simulink model "FireFighter_original"  (R2014a)
settings: Solver=ode45  StartTime=0.0  StopTime=150  RelTol=1e-3
undefined symbols (not defined in the file): DiscIntNeverNeededParam, sigbuilder_block
libraries: simulink x68
(part 2 of 6)

== system FireFighter_original/FF_Signals4/Environment1 ==
  note: F_hill
  note: F_eng_resistance
  note: F_resistance
  note: F_eng
  note: position
  note: speed
  note: slope
  gas : Inport
  brake : Inport  Port=2
  1/mass2 : Gain  Gain=0.001
  Discrete-Time Integrator : DiscreteIntegrator  SampleTime=-1  ICPrevOutput=DiscIntNeverNeededParam  ICPrevScaledInput=DiscIntNeverNeededParam
  Discrete-Time Integrator1 : DiscreteIntegrator  SampleTime=-1  ICPrevOutput=DiscIntNeverNeededParam  ICPrevScaledInput=DiscIntNeverNeededParam
  Fast - to - Slow : RateTransition  OutPortSampleTimeMultiple=0.05  OutPortSampleTime=0.1
  "Fast - to - Slow1 " : RateTransition  OutPortSampleTimeMultiple=0.05  OutPortSampleTime=0.1
  Fcn : Fcn  Expr=u(1)/0.005
  Gain1 : Gain  Gain=0.0005
  Max Torque by rpm6 : Lookup_n-D  NumberOfTableDimensions=1  BreakpointsForDimension1=[0;8;20;28;40;60;80;100;120;140;160;180;200]  Table=[165;180;180;170;170;150;115;97;80;70;60;50;40]  RndMeth=Simplest  InputSameDT=on
  Max Torque by rpm9 : Lookup_n-D  NumberOfTableDimensions=1  BreakpointsForDimension1=[0:1000:15000]  Table=[0;pi/60;pi/30;pi/20;pi/15;pi/12;0;0;-pi/18;-pi/36;0;0;0;0;0;0]  RndMeth=Simplest  InputSameDT=on
  Product1 : Product  RndMeth=Zero
  Scope{2..3,6..15,27} (13 alike) : Scope
      Scope10 settings: SaveName=ScopeData23
      Scope11 settings: TimeRange=10  YMin=-50  YMax=300  SaveName=ScopeData26
      Scope12 settings: SaveName=ScopeData32
      Scope13 settings: SaveName=ScopeData33
      Scope14 settings: SaveName=ScopeData15
      Scope15 settings: SaveName=ScopeData19
      Scope2 settings: TimeRange=10  YMin=-50  YMax=300  SaveName=ScopeData6
      Scope27 settings: TimeRange=10  YMin=-50  YMax=300  SaveName=ScopeData49
      Scope3 settings: SaveName=ScopeData8
      Scope6 settings: TimeRange=100  YMin=89.9904  YMax=89.9913  SaveName=ScopeData16
      Scope7 settings: SaveName=ScopeData10
      Scope8 settings: SaveName=ScopeData21
      Scope9 settings: SaveName=ScopeData22
  Slow - to - Fast : RateTransition  OutPortSampleTimeMultiple=0.05  OutPortSampleTime=0.05
  Step1 : Step  Time=0  After=700
  Sum1 : Sum  Inputs=|++
  Sum4 : Sum  Inputs=|+---
  Trigonometric Function1 : Trigonometry
  brake force1 : Gain  Gain=10000
  g1 : Gain  Gain=9.80665
  mass3 : Gain  Gain=1000
  pos : Outport
  wires:
  Step1/1 -> Sum1/2
  Product1/1 -> Fcn/1
  brake force1/1 -> Scope12/1, Sum4/2
  Sum4/1 -> Scope7/1, 1/mass2/1
  1/mass2/1 -> Discrete-Time Integrator/1, Scope8/1
  Gain1/1 -> Scope13/1, Sum4/3
  gas/1 -> Scope14/1, Fast - to - Slow/1
  brake/1 -> Scope15/1, "Fast - to - Slow1 "/1
  Discrete-Time Integrator/1 -> Max Torque by rpm6/1, Gain1/1, Discrete-Time Integrator1/1, Scope6/1
  Discrete-Time Integrator1/1 -> Max Torque by rpm9/1, Scope2/1, Sum1/1
  Max Torque by rpm9/1 -> Trigonometric Function1/1
  g1/1 -> mass3/1
  Trigonometric Function1/1 -> g1/1
  mass3/1 -> Sum4/4, Scope3/1
  Fcn/1 -> Scope10/1, Sum4/1
  Fast - to - Slow/1 -> Product1/2
  "Fast - to - Slow1 "/1 -> brake force1/1
  Sum1/1 -> Scope27/1, Slow - to - Fast/1
  Slow - to - Fast/1 -> pos/1, Scope11/1
  Max Torque by rpm6/1 -> Product1/1, Scope9/1

== system FireFighter_original/FF_Signals4/FireFighter1 ==
  note: current speed
  note: speed=90
  pos : Inport
  Constant : Constant  Value=0
  Constant2 : Constant  Value=90
  Discrete Derivative : simulink/Discrete/Discrete Derivative  gainval=1.0  ICPrevScaledInput=0.0  InputProcessing=Inherited  OutMin=[]  OutMax=[]  OutDataType=fixdt(1, 16)  OutScaling=2^-10  DoSatur=off
  Discrete PID Controller : simulink/Continuous/PID Controller  Controller=PI  TimeDomain=Discrete-time  SampleTime=-1  IntegratorMethod=Forward Euler  FilterMethod=Forward Euler  Form=Parallel  P=0.05  I=0.000228325  D=0  N=100  InitialConditionSource=internal  InitialConditionForIntegrator=0  InitialConditionForFilter=0  ExternalReset=none  LimitOutput=on  UpperSaturationLimit=1  LowerSaturationLimit=-1  LinearizeAsGain=off  AntiWindupMode=back-calculation  Kb=0.01  TrackingMode=off  Kt=1  PParamMin=[]  PParamMax=[]  IParamMin=[]  IParamMax=[]  DParamMin=[]  DParamMax=[]  NParamMin=[]  NParamMax=[]  KbParamMin=[]  KbParamMax=[]  KtParamMin=[]  KtParamMax=[]  POutMin=[]  POutMax=[]  IOutMin=[]  IOutMax=[]  DOutMin=[]  DOutMax=[]  NOutMin=[]  NOutMax=[]  KbOutMin=[]  KbOutMax=[]  KtOutMin=[]  KtOutMax=[]  IntegratorOutMin=[]  IntegratorOutMax=[]  FilterOutMin=[]  FilterOutMax=[]  SumOutMin=[]  SumOutMax=[]  SumI1OutMin=[]  SumI1OutMax=[]  SumI2OutMin=[]  SumI2OutMax=[]  SumI3OutMin=[]  SumI3OutMax=[]  SumDOutMin=[]  SumDOutMax=[]  SaturationOutMin=[]  SaturationOutMax=[]  IntegratorContinuousStateAttributes=''  IntegratorStateMustResolveToSignalObject=off  IntegratorRTWStateStorageClass=Auto  FilterContinuousStateAttributes=''  FilterStateMustResolveToSignalObject=off  FilterRTWStateStorageClass=Auto
  Fast - to -Slow : RateTransition  OutPortSampleTimeMultiple=0.05  OutPortSampleTime=0.1
  Gain : Gain  Gain=50
  Gain1 : Gain  Gain=-1
  Scope{1..2,4..9,11..13} (11 alike) : Scope
      Scope1 settings: TimeRange=100  YMin=90  YMax=130
      Scope11 settings: YMin=-300  YMax=300  SaveName=ScopeData28
      Scope12 settings: YMin=-300  YMax=300  SaveName=ScopeData30
      Scope13 settings: SaveName=ScopeData31
      Scope2 settings: YMin=-300  YMax=300  SaveName=ScopeData2
      Scope4 settings: YMin=-300  YMax=300  SaveName=ScopeData17
      Scope5 settings: SaveName=ScopeData20
      Scope6 settings: YMin=-300  YMax=300  SaveName=ScopeData18
      Scope7 settings: YMin=-300  YMax=300  SaveName=ScopeData24
      Scope8 settings: TimeRange=10  SaveName=ScopeData25
      Scope9 settings: SaveName=ScopeData38
  Signal Builder : Subsystem  Tag=STV Subsys  LoadFcn=sigbuilder_block('load');  StartFcn=sigbuilder_block('start');  StopFcn=sigbuilder_block('stop');  ClipboardFcn=sigbuilder_block('clipboard');  mask(Sigbuilder block){}
      mask help: Simulink:masks:SigbuilderBlock_MD
      mask init:
      | if ~strcmp(get_param(bdroot(gcbh),'SimulationStatus'),'stopped') tuvar = sigbuilder_block('maskInit'); end
      settings: CopyFcn=sigbuilder_block('copy');  DeleteFcn=sigbuilder_block('delete');  ModelCloseFcn=sigbuilder_block('modelClose');  PreSaveFcn=sigbuilder_block('preSave');  PauseFcn=sigbuilder_block('pause');  ContinueFcn=sigbuilder_block('continue');  NameChangeFcn=sigbuilder_block('namechange');  OpenFcn=sigbuilder_block('open',[359.25 300.75 550.5 399.75 ]);  CloseFcn=sigbuilder_block('close');
      mask Display: plot(0, 0, 100, 100,[2, 2, 32, 32, 2], [68, 8, 8, 68, 68],[32, 2], [38, 38], [32, 19, 2],[53, 60, 44], [32, 17, 17, 2],[16, 16, 31, 31]);txt = getActiveGroup(gcbh);text(2, 100, txt,'verticalAlignment', 'top');
  Slow - to - Fast : RateTransition  OutPortSampleTimeMultiple=0.05  OutPortSampleTime=0.05
  Slow - to - Fast1 : RateTransition  OutPortSampleTimeMultiple=0.05  OutPortSampleTime=0.05
  Sum : Sum  Inputs=|+-
  Sum1 : Sum  Inputs=|++
  Switch : Switch
  Switch1 : Switch
  Zero-Order Hold : ZeroOrderHold  SampleTime=0.1
  gas : Outport
  brake : Outport  Port=2
  wires:
  Discrete Derivative/1 -> Scope8/1, Sum/2
  Signal Builder/1(Signal 1) -> Gain/1
  Gain/1 -> Zero-Order Hold/1
  Constant2/1 -> Sum1/2
  Discrete PID Controller/1 -> Scope2/1, Scope7/1, Switch/1, Switch/2, Switch1/2, Gain1/1
  Gain1/1 -> Switch1/3
  Switch/1 -> Slow - to - Fast/1, Scope4/1
  Constant/1 -> Switch/3, Switch1/1
  Switch1/1 -> Slow - to - Fast1/1, Scope6/1
  pos/1 -> Scope13/1, Fast - to -Slow/1
  Sum/1 -> Discrete PID Controller/1, Scope9/1
  Fast - to -Slow/1 -> Discrete Derivative/1, Scope5/1
  Slow - to - Fast/1 -> Scope11/1, gas/1
  Slow - to - Fast1/1 -> Scope12/1, brake/1
  Sum1/1 -> Scope1/1, Sum/1
  Zero-Order Hold/1 -> Sum1/1

== system FireFighter_original/FF_Signals4/Inaccuracy ==
  note: max
  pos_init : Inport
  hold : Inport  Port=2
  Mux29 : Mux  Inputs=2
  Product : Product
  Product1 : Product
  Scope{1..3,5..7,9} (7 alike) : Scope
      Scope1 settings: SaveName=ScopeData29
      Scope2 settings: SaveName=ScopeData43
      Scope3 settings: SaveName=ScopeData35
      Scope5 settings: SaveName=ScopeData46
      Scope6 settings: SaveName=ScopeData48
      Scope7 settings: TimeRange=150  SaveName=ScopeData57
      Scope9 settings: SaveName=ScopeData44
  Subsystem1 : Subsystem
  Subsystem2 : Subsystem
  Subtract1 : Sum  Inputs=-+
  result : Outport
  wires:
  Subsystem2/1(min) -> Product/1, Scope2/1  "min"
  pos_init/1 -> Subsystem1/1(pos_init), Subsystem2/1(pos_init), Scope1/1
  Mux29/1 -> result/1
  Subsystem1/1(max) -> Product1/2, Scope9/1
  Product/1 -> Mux29/1, Scope6/1, Subtract1/1
  Product1/1 -> Scope5/1, Mux29/2, Subtract1/2
  hold/1 -> Subsystem2/2(hold), Scope3/1, Product/2, Product1/1, Subsystem1/2(hold)
  Subtract1/1 -> Scope7/1

== system FireFighter_original/FF_Signals4/Inaccuracy1 ==
  note: max
  Hpos_inits : Inport
  holds : Inport  Port=2
  Mux29 : Mux  Inputs=2
  Product : Product
  Product1 : Product
  Scope{1..3,5..7,9} (7 alike) : Scope
      Scope1 settings: SaveName=ScopeData29
      Scope2 settings: SaveName=ScopeData43
      Scope3 settings: SaveName=ScopeData35
      Scope5 settings: SaveName=ScopeData46
      Scope6 settings: SaveName=ScopeData48
      Scope7 settings: TimeRange=150  SaveName=ScopeData57
      Scope9 settings: SaveName=ScopeData44
  Subsystem1 : Subsystem
  Subsystem2 : Subsystem
  Subtract1 : Sum  Inputs=-+
  result : Outport
  wires:
  Subsystem2/1(min) -> Product/1, Scope2/1  "min"
  Hpos_inits/1 -> Subsystem1/1(pos_init), Subsystem2/1(pos_init), Scope1/1
  Mux29/1 -> result/1
  Subsystem1/1(max) -> Product1/2, Scope9/1
  Product/1 -> Mux29/1, Scope6/1, Subtract1/1
  Product1/1 -> Scope5/1, Mux29/2, Subtract1/2
  holds/1 -> Subsystem2/2(hold), Scope3/1, Product/2, Product1/1, Subsystem1/2(hold)
  Subtract1/1 -> Scope7/1

== system FireFighter_original/FF_Signals4/Inaccuracy2 ==
  note: max
  Hpos_inits : Inport
  holds : Inport  Port=2
  Mux29 : Mux  Inputs=2
  Product : Product
  Product1 : Product
  Scope{1..3,5..7,9} (7 alike) : Scope
      Scope1 settings: SaveName=ScopeData29
      Scope2 settings: SaveName=ScopeData43
      Scope3 settings: SaveName=ScopeData35
      Scope5 settings: SaveName=ScopeData46
      Scope6 settings: SaveName=ScopeData48
      Scope7 settings: TimeRange=150  SaveName=ScopeData57
      Scope9 settings: SaveName=ScopeData44
  Subsystem1 : Subsystem
  Subsystem2 : Subsystem
  Subtract1 : Sum  Inputs=-+
  result : Outport
  wires:
  Subsystem2/1(min) -> Product/1, Scope2/1  "min"
  Hpos_inits/1 -> Subsystem1/1(pos_init), Subsystem2/1(pos_init), Scope1/1
  Mux29/1 -> result/1
  Subsystem1/1(max) -> Product1/2, Scope9/1
  Product/1 -> Mux29/1, Scope6/1, Subtract1/1
  Product1/1 -> Scope5/1, Mux29/2, Subtract1/2
  holds/1 -> Subsystem2/2(hold), Scope3/1, Product/2, Product1/1, Subsystem1/2(hold)
  Subtract1/1 -> Scope7/1

== system FireFighter_original/FF_Signals4/START THE MESSION2 ==
  Demux : Demux  Tag=STV Demux  Outputs=1
  FromWs : FromWorkspace  Tag=STV FromWs  VariableName=tuvar  SampleTime=0
      SigBuilderData=|
      | common.afterFinalStr = 'Extrapolate'
      | common.sampleTime = 0
      | dataSet.timeRange = [0 1000]
      | dataSet.name = 'Group 1'
      | sbobj.Groups.Name = 'Group 1'
      | sbobj.Groups.Signals.Name = 'SWITCH'
      | sbobj.Groups.Signals.XData = [0 20 20 1000]
      | sbobj.Groups.Signals.YData = [0 0 1 1]
      | sbobj.Groups.TimeRange = [0 1000]
  SWITCH : Outport  Tag=STV Outport
  wires:
  FromWs/1 -> Demux/1
  Demux/1 -> SWITCH/1

== system FireFighter_original/Inaccuracy/Subsystem1 ==
  pos_init : Inport
  hold : Inport  Port=2
  Environment : Subsystem
  FireFighter : Subsystem
  max : Outport
  wires:
  Environment/1(pos) -> FireFighter/1(pos), max/1
  FireFighter/1(gas) -> Environment/1(gas)
  FireFighter/2(brake) -> Environment/2(brake)
  pos_init/1 -> Environment/3(pos_init)
  hold/1 -> Environment/4(hold)

== system FireFighter_original/Inaccuracy/Subsystem2 ==
  pos_init : Inport
  hold : Inport  Port=2
  Environment : Subsystem
  FireFighter : Subsystem
  min : Outport
  wires:
  Environment/1(pos) -> FireFighter/1(pos), min/1
  FireFighter/1(gas) -> Environment/1(gas)
  FireFighter/2(brake) -> Environment/2(brake)
  pos_init/1 -> Environment/3(pos_init)
  hold/1 -> Environment/4(hold)

== system FireFighter_original/FF_Signals/FireFighter/Signal Builder ==
  Demux : Demux  Tag=STV Demux  Outputs=1
  FromWs : FromWorkspace  Tag=STV FromWs  VariableName=tuvar  SampleTime=0
      SigBuilderData=|
      | common.afterFinalStr = 'Extrapolate'
      | common.sampleTime = 0
      | dataSet.timeRange = [0 100]
      | dataSet.name = 'Group 1'
      | sbobj.Groups.Name = 'Group 1'
      | sbobj.Groups.Signals.Name = 'Signal 1'
      | sbobj.Groups.Signals.XData = [0 30 40 50 70 100]
      | sbobj.Groups.Signals.YData = [0 0 0.6 -0.405 0 0]
      | sbobj.Groups.TimeRange = [0 100]
  Signal 1 : Outport  Tag=STV Outport
  wires:
  Demux/1 -> Signal 1/1
  FromWs/1 -> Demux/1

== system FireFighter_original/FF_Signals1/FireFighter1/Signal Builder ==
  Demux : Demux  Tag=STV Demux  Outputs=1
  FromWs : FromWorkspace  Tag=STV FromWs  VariableName=tuvar  SampleTime=0
      SigBuilderData=|
      | common.afterFinalStr = 'Extrapolate'
      | common.sampleTime = 0
      | dataSet.timeRange = [0 100]
      | dataSet.name = 'Group 1'
      | sbobj.Groups.Name = 'Group 1'
      | sbobj.Groups.Signals.Name = 'Signal 1'
      | sbobj.Groups.Signals.XData = [0 30 40 50 70 100]
      | sbobj.Groups.Signals.YData = [0 0 0.6 -0.405 0 0]
      | sbobj.Groups.TimeRange = [0 100]
  Signal 1 : Outport  Tag=STV Outport
  wires:
  Demux/1 -> Signal 1/1
  FromWs/1 -> Demux/1

== system FireFighter_original/FF_Signals1/Inaccuracy/Subsystem1 ==
  pos_init : Inport
  hold : Inport  Port=2
  Environment : Subsystem
  FireFighter : Subsystem
  max : Outport
  wires:
  Environment/1(pos) -> FireFighter/1(pos), max/1
  FireFighter/1(gas) -> Environment/1(gas)
  FireFighter/2(brake) -> Environment/2(brake)
  pos_init/1 -> Environment/3(pos_init)
  hold/1 -> Environment/4(hold)

== system FireFighter_original/FF_Signals1/Inaccuracy/Subsystem2 ==
  pos_init : Inport
  hold : Inport  Port=2
  Environment : Subsystem
  FireFighter : Subsystem
  min : Outport
  wires:
  Environment/1(pos) -> FireFighter/1(pos), min/1
  FireFighter/1(gas) -> Environment/1(gas)
  FireFighter/2(brake) -> Environment/2(brake)
  pos_init/1 -> Environment/3(pos_init)
  hold/1 -> Environment/4(hold)

== system FireFighter_original/FF_Signals1/Inaccuracy1/Subsystem1 ==
  pos_init : Inport
  hold : Inport  Port=2
  Environment : Subsystem
  FireFighter : Subsystem
  max : Outport
  wires:
  Environment/1(pos) -> FireFighter/1(pos), max/1
  FireFighter/1(gas) -> Environment/1(gas)
  FireFighter/2(brake) -> Environment/2(brake)
  pos_init/1 -> Environment/3(pos_init)
  hold/1 -> Environment/4(hold)

== system FireFighter_original/FF_Signals1/Inaccuracy1/Subsystem2 ==
  pos_init : Inport
  hold : Inport  Port=2
  Environment : Subsystem
  FireFighter : Subsystem
  min : Outport
  wires:
  Environment/1(pos) -> FireFighter/1(pos), min/1
  FireFighter/1(gas) -> Environment/1(gas)
  FireFighter/2(brake) -> Environment/2(brake)
  pos_init/1 -> Environment/3(pos_init)
  hold/1 -> Environment/4(hold)

== system FireFighter_original/FF_Signals1/Inaccuracy2/Subsystem1 ==
  pos_init : Inport
  hold : Inport  Port=2
  Environment : Subsystem
  FireFighter : Subsystem
  max : Outport
  wires:
  Environment/1(pos) -> FireFighter/1(pos), max/1
  FireFighter/1(gas) -> Environment/1(gas)
  FireFighter/2(brake) -> Environment/2(brake)
  pos_init/1 -> Environment/3(pos_init)
  hold/1 -> Environment/4(hold)

== system FireFighter_original/FF_Signals1/Inaccuracy2/Subsystem2 ==
  pos_init : Inport
  hold : Inport  Port=2
  Environment : Subsystem
  FireFighter : Subsystem
  min : Outport
  wires:
  Environment/1(pos) -> FireFighter/1(pos), min/1
  FireFighter/1(gas) -> Environment/1(gas)
  FireFighter/2(brake) -> Environment/2(brake)
  pos_init/1 -> Environment/3(pos_init)
  hold/1 -> Environment/4(hold)

== system FireFighter_original/FF_Signals2/FireFighter1/Signal Builder ==
  Demux : Demux  Tag=STV Demux  Outputs=1
  FromWs : FromWorkspace  Tag=STV FromWs  VariableName=tuvar  SampleTime=0
      SigBuilderData=|
      | common.afterFinalStr = 'Extrapolate'
      | common.sampleTime = 0
      | dataSet.timeRange = [0 100]
      | dataSet.name = 'Group 1'
      | sbobj.Groups.Name = 'Group 1'
      | sbobj.Groups.Signals.Name = 'Signal 1'
      | sbobj.Groups.Signals.XData = [0 30 40 50 70 100]
      | sbobj.Groups.Signals.YData = [0 0 0.6 -0.405 0 0]
      | sbobj.Groups.TimeRange = [0 100]
  Signal 1 : Outport  Tag=STV Outport
  wires:
  Demux/1 -> Signal 1/1
  FromWs/1 -> Demux/1

== system FireFighter_original/FF_Signals2/Inaccuracy/Subsystem1 ==
  pos_init : Inport
  hold : Inport  Port=2
  Environment : Subsystem
  FireFighter : Subsystem
  max : Outport
  wires:
  Environment/1(pos) -> FireFighter/1(pos), max/1
  FireFighter/1(gas) -> Environment/1(gas)
  FireFighter/2(brake) -> Environment/2(brake)
  pos_init/1 -> Environment/3(pos_init)
  hold/1 -> Environment/4(hold)

== system FireFighter_original/FF_Signals2/Inaccuracy/Subsystem2 ==
  pos_init : Inport
  hold : Inport  Port=2
  Environment : Subsystem
  FireFighter : Subsystem
  min : Outport
  wires:
  Environment/1(pos) -> FireFighter/1(pos), min/1
  FireFighter/1(gas) -> Environment/1(gas)
  FireFighter/2(brake) -> Environment/2(brake)
  pos_init/1 -> Environment/3(pos_init)
  hold/1 -> Environment/4(hold)

== system FireFighter_original/FF_Signals2/Inaccuracy1/Subsystem1 ==
  pos_init : Inport
  hold : Inport  Port=2
  Environment : Subsystem
  FireFighter : Subsystem
  max : Outport
  wires:
  Environment/1(pos) -> FireFighter/1(pos), max/1
  FireFighter/1(gas) -> Environment/1(gas)
  FireFighter/2(brake) -> Environment/2(brake)
  pos_init/1 -> Environment/3(pos_init)
  hold/1 -> Environment/4(hold)

== system FireFighter_original/FF_Signals2/Inaccuracy1/Subsystem2 ==
  pos_init : Inport
  hold : Inport  Port=2
  Environment : Subsystem
  FireFighter : Subsystem
  min : Outport
  wires:
  Environment/1(pos) -> FireFighter/1(pos), min/1
  FireFighter/1(gas) -> Environment/1(gas)
  FireFighter/2(brake) -> Environment/2(brake)
  pos_init/1 -> Environment/3(pos_init)
  hold/1 -> Environment/4(hold)

== system FireFighter_original/FF_Signals2/Inaccuracy2/Subsystem1 ==
  pos_init : Inport
  hold : Inport  Port=2
  Environment : Subsystem
  FireFighter : Subsystem
  max : Outport
  wires:
  Environment/1(pos) -> FireFighter/1(pos), max/1
  FireFighter/1(gas) -> Environment/1(gas)
  FireFighter/2(brake) -> Environment/2(brake)
  pos_init/1 -> Environment/3(pos_init)
  hold/1 -> Environment/4(hold)

== system FireFighter_original/FF_Signals2/Inaccuracy2/Subsystem2 ==
  pos_init : Inport
  hold : Inport  Port=2
  Environment : Subsystem
  FireFighter : Subsystem
  min : Outport
  wires:
  Environment/1(pos) -> FireFighter/1(pos), min/1
  FireFighter/1(gas) -> Environment/1(gas)
  FireFighter/2(brake) -> Environment/2(brake)
  pos_init/1 -> Environment/3(pos_init)
  hold/1 -> Environment/4(hold)

== system FireFighter_original/FF_Signals4/FireFighter1/Signal Builder ==
  Demux : Demux  Tag=STV Demux  Outputs=1
  FromWs : FromWorkspace  Tag=STV FromWs  VariableName=tuvar  SampleTime=0
      SigBuilderData=|
      | common.afterFinalStr = 'Extrapolate'
      | common.sampleTime = 0
      | dataSet.timeRange = [0 100]
      | dataSet.name = 'Group 1'
      | sbobj.Groups.Name = 'Group 1'
      | sbobj.Groups.Signals.Name = 'Signal 1'
      | sbobj.Groups.Signals.XData = [0 30 40 50 70 100]
      | sbobj.Groups.Signals.YData = [0 0 0.6 -0.405 0 0]
      | sbobj.Groups.TimeRange = [0 100]
  Signal 1 : Outport  Tag=STV Outport
  wires:
  Demux/1 -> Signal 1/1
  FromWs/1 -> Demux/1

== system FireFighter_original/FF_Signals4/Inaccuracy/Subsystem1 ==
  pos_init : Inport
  hold : Inport  Port=2
  Environment : Subsystem
  FireFighter : Subsystem
  max : Outport
  wires:
  Environment/1(pos) -> FireFighter/1(pos), max/1
  FireFighter/1(gas) -> Environment/1(gas)
  FireFighter/2(brake) -> Environment/2(brake)
  pos_init/1 -> Environment/3(pos_init)
  hold/1 -> Environment/4(hold)

== system FireFighter_original/FF_Signals4/Inaccuracy/Subsystem2 ==
  pos_init : Inport
  hold : Inport  Port=2
  Environment : Subsystem
  FireFighter : Subsystem
  min : Outport
  wires:
  Environment/1(pos) -> FireFighter/1(pos), min/1
  FireFighter/1(gas) -> Environment/1(gas)
  FireFighter/2(brake) -> Environment/2(brake)
  pos_init/1 -> Environment/3(pos_init)
  hold/1 -> Environment/4(hold)

== system FireFighter_original/FF_Signals4/Inaccuracy1/Subsystem1 ==
  pos_init : Inport
  hold : Inport  Port=2
  Environment : Subsystem
  FireFighter : Subsystem
  max : Outport
  wires:
  Environment/1(pos) -> FireFighter/1(pos), max/1
  FireFighter/1(gas) -> Environment/1(gas)
  FireFighter/2(brake) -> Environment/2(brake)
  pos_init/1 -> Environment/3(pos_init)
  hold/1 -> Environment/4(hold)

== system FireFighter_original/FF_Signals4/Inaccuracy1/Subsystem2 ==
  pos_init : Inport
  hold : Inport  Port=2
  Environment : Subsystem
  FireFighter : Subsystem
  min : Outport
  wires:
  Environment/1(pos) -> FireFighter/1(pos), min/1
  FireFighter/1(gas) -> Environment/1(gas)
  FireFighter/2(brake) -> Environment/2(brake)
  pos_init/1 -> Environment/3(pos_init)
  hold/1 -> Environment/4(hold)

== system FireFighter_original/FF_Signals4/Inaccuracy2/Subsystem1 ==
  pos_init : Inport
  hold : Inport  Port=2
  Environment : Subsystem
  FireFighter : Subsystem
  max : Outport
  wires:
  Environment/1(pos) -> FireFighter/1(pos), max/1
  FireFighter/1(gas) -> Environment/1(gas)
  FireFighter/2(brake) -> Environment/2(brake)
  pos_init/1 -> Environment/3(pos_init)
  hold/1 -> Environment/4(hold)

== system FireFighter_original/FF_Signals4/Inaccuracy2/Subsystem2 ==
  pos_init : Inport
  hold : Inport  Port=2
  Environment : Subsystem
  FireFighter : Subsystem
  min : Outport
  wires:
  Environment/1(pos) -> FireFighter/1(pos), min/1
  FireFighter/1(gas) -> Environment/1(gas)
  FireFighter/2(brake) -> Environment/2(brake)
  pos_init/1 -> Environment/3(pos_init)
  hold/1 -> Environment/4(hold)

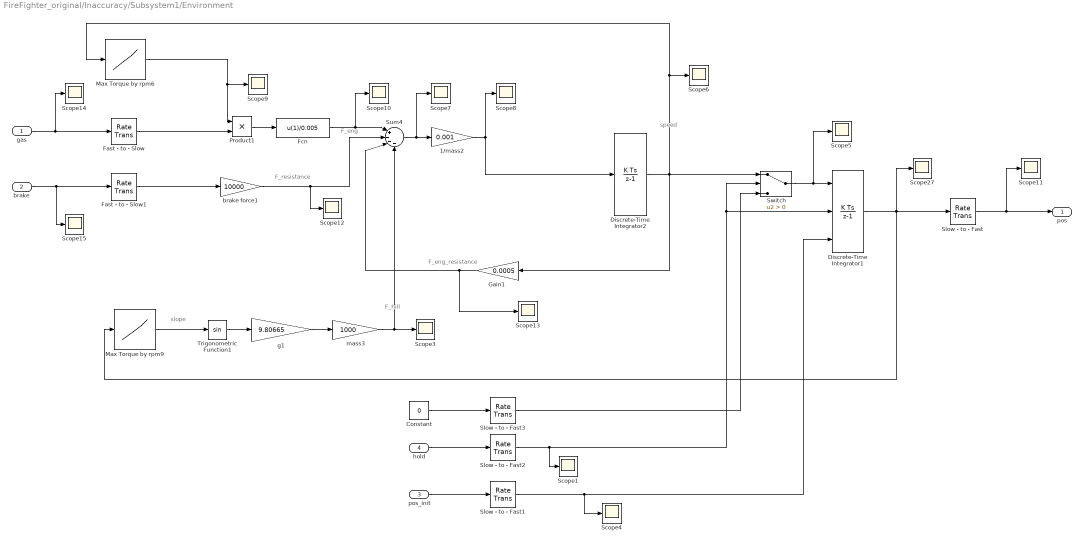
== system FireFighter_original/Inaccuracy/Subsystem1/Environment ==
  note: F_hill
  note: F_eng_resistance
  note: F_resistance
  note: F_eng
  note: slope
  note: speed
  gas : Inport
  brake : Inport  Port=2
  pos_init : Inport  Port=3
  hold : Inport  Port=4
  1/mass2 : Gain  Gain=0.001
  Constant : Constant  Value=0
  Discrete-Time Integrator1 : DiscreteIntegrator  ExternalReset=rising  InitialConditionSource=external  SampleTime=-1  ICPrevOutput=DiscIntNeverNeededParam  ICPrevScaledInput=DiscIntNeverNeededParam
  Discrete-Time Integrator2 : DiscreteIntegrator  SampleTime=-1  ICPrevOutput=DiscIntNeverNeededParam  ICPrevScaledInput=DiscIntNeverNeededParam
  Fast - to - Slow : RateTransition  OutPortSampleTimeMultiple=0.05  OutPortSampleTime=0.1
  "Fast - to - Slow1 " : RateTransition  OutPortSampleTimeMultiple=0.05  OutPortSampleTime=0.1
  Fcn : Fcn  Expr=u(1)/0.005
  Gain1 : Gain  Gain=0.0005
  Max Torque by rpm6 : Lookup_n-D  NumberOfTableDimensions=1  BreakpointsForDimension1=[0;8;20;28;40;60;80;100;120;140;160;180;200]  Table=[165;180;180;170;170;150;115;97;80;70;60;50;40]  RndMeth=Simplest  InputSameDT=on
  Max Torque by rpm9 : Lookup_n-D  NumberOfTableDimensions=1  BreakpointsForDimension1=[0:1000:15000]  Table=[0;pi/60;pi/30;pi/20;pi/15;pi/12;0;0;-pi/18;-pi/36;0;0;0;0;0;0]  RndMeth=Simplest  InputSameDT=on
  Product1 : Product  RndMeth=Zero
  Scope{1,3..15,27} (15 alike) : Scope
      Scope1 settings: TimeRange=10  YMin=-50  YMax=300  SaveName=ScopeData51
      Scope10 settings: SaveName=ScopeData23
      Scope11 settings: TimeRange=10  YMin=-50  YMax=300  SaveName=ScopeData26
      Scope12 settings: SaveName=ScopeData32
      Scope13 settings: SaveName=ScopeData33
      Scope14 settings: SaveName=ScopeData15
      Scope15 settings: SaveName=ScopeData19
      Scope27 settings: TimeRange=10  YMin=-50  YMax=300  SaveName=ScopeData49
      Scope3 settings: SaveName=ScopeData8
      Scope4 settings: TimeRange=10  YMin=-50  YMax=300  SaveName=ScopeData53
      Scope5 settings: TimeRange=10  YMin=-50  YMax=300  SaveName=ScopeData54
      Scope6 settings: TimeRange=100  YMin=0  YMax=300  SaveName=ScopeData55
      Scope7 settings: SaveName=ScopeData10
      Scope8 settings: SaveName=ScopeData21
      Scope9 settings: SaveName=ScopeData22
  Slow - to - Fast{,1..3} (4 alike) : RateTransition  OutPortSampleTimeMultiple=0.05  OutPortSampleTime=0.05
  Sum4 : Sum  Inputs=|+---
  Switch : Switch  Criteria=u2 > Threshold
  Trigonometric Function1 : Trigonometry
  brake force1 : Gain  Gain=10000
  g1 : Gain  Gain=9.80665
  mass3 : Gain  Gain=1000
  pos : Outport
  wires:
  Product1/1 -> Fcn/1
  brake force1/1 -> Scope12/1, Sum4/2
  Sum4/1 -> Scope7/1, 1/mass2/1
  1/mass2/1 -> Discrete-Time Integrator2/1, Scope8/1
  Gain1/1 -> Scope13/1, Sum4/3
  gas/1 -> Scope14/1, Fast - to - Slow/1
  brake/1 -> Scope15/1, "Fast - to - Slow1 "/1
  Max Torque by rpm9/1 -> Trigonometric Function1/1
  g1/1 -> mass3/1
  Trigonometric Function1/1 -> g1/1
  mass3/1 -> Sum4/4, Scope3/1
  Fcn/1 -> Scope10/1, Sum4/1
  Fast - to - Slow/1 -> Product1/2
  "Fast - to - Slow1 "/1 -> brake force1/1
  Slow - to - Fast/1 -> pos/1, Scope11/1
  Max Torque by rpm6/1 -> Product1/1, Scope9/1
  Discrete-Time Integrator2/1 -> Max Torque by rpm6/1, Scope6/1, Switch/1, Gain1/1
  pos_init/1 -> Slow - to - Fast1/1
  hold/1 -> Slow - to - Fast2/1
  Slow - to - Fast2/1 -> Switch/2, Discrete-Time Integrator1/2, Scope1/1
  Slow - to - Fast1/1 -> Scope4/1, Discrete-Time Integrator1/3
  Constant/1 -> Slow - to - Fast3/1
  Slow - to - Fast3/1 -> Switch/3
  Discrete-Time Integrator1/1 -> Max Torque by rpm9/1, Scope27/1, Slow - to - Fast/1
  Switch/1 -> Scope5/1, Discrete-Time Integrator1/1

== system FireFighter_original/Inaccuracy/Subsystem1/FireFighter ==
  note: current speed
  note: speed=90
  pos : Inport
  Constant : Constant  Value=0
  Constant1 : Constant  Value=250
  Constant2 : Constant  Value=250
  Discrete Derivative : simulink/Discrete/Discrete Derivative  gainval=1.0  ICPrevScaledInput=0.0  InputProcessing=Inherited  OutMin=[]  OutMax=[]  OutDataType=fixdt(1, 16)  OutScaling=2^-10  DoSatur=off
  Discrete PID Controller : simulink/Continuous/PID Controller  Controller=PI  TimeDomain=Discrete-time  SampleTime=-1  IntegratorMethod=Forward Euler  FilterMethod=Forward Euler  Form=Parallel  P=0.05  I=0.000228325  D=0  N=100  InitialConditionSource=internal  InitialConditionForIntegrator=0  InitialConditionForFilter=0  ExternalReset=none  LimitOutput=on  UpperSaturationLimit=1  LowerSaturationLimit=-1  LinearizeAsGain=off  AntiWindupMode=back-calculation  Kb=0.01  TrackingMode=off  Kt=1  PParamMin=[]  PParamMax=[]  IParamMin=[]  IParamMax=[]  DParamMin=[]  DParamMax=[]  NParamMin=[]  NParamMax=[]  KbParamMin=[]  KbParamMax=[]  KtParamMin=[]  KtParamMax=[]  POutMin=[]  POutMax=[]  IOutMin=[]  IOutMax=[]  DOutMin=[]  DOutMax=[]  NOutMin=[]  NOutMax=[]  KbOutMin=[]  KbOutMax=[]  KtOutMin=[]  KtOutMax=[]  IntegratorOutMin=[]  IntegratorOutMax=[]  FilterOutMin=[]  FilterOutMax=[]  SumOutMin=[]  SumOutMax=[]  SumI1OutMin=[]  SumI1OutMax=[]  SumI2OutMin=[]  SumI2OutMax=[]  SumI3OutMin=[]  SumI3OutMax=[]  SumDOutMin=[]  SumDOutMax=[]  SaturationOutMin=[]  SaturationOutMax=[]  IntegratorContinuousStateAttributes=''  IntegratorStateMustResolveToSignalObject=off  IntegratorRTWStateStorageClass=Auto  FilterContinuousStateAttributes=''  FilterStateMustResolveToSignalObject=off  FilterRTWStateStorageClass=Auto
  Discrete PID Controller1 : simulink/Continuous/PID Controller  Controller=PI  TimeDomain=Discrete-time  SampleTime=-1  IntegratorMethod=Forward Euler  FilterMethod=Forward Euler  Form=Parallel  P=0.05  I=0.000228325  D=0  N=100  InitialConditionSource=internal  InitialConditionForIntegrator=0  InitialConditionForFilter=0  ExternalReset=none  LimitOutput=on  UpperSaturationLimit=1  LowerSaturationLimit=-1  LinearizeAsGain=off  AntiWindupMode=back-calculation  Kb=0.01  TrackingMode=off  Kt=1  PParamMin=[]  PParamMax=[]  IParamMin=[]  IParamMax=[]  DParamMin=[]  DParamMax=[]  NParamMin=[]  NParamMax=[]  KbParamMin=[]  KbParamMax=[]  KtParamMin=[]  KtParamMax=[]  POutMin=[]  POutMax=[]  IOutMin=[]  IOutMax=[]  DOutMin=[]  DOutMax=[]  NOutMin=[]  NOutMax=[]  KbOutMin=[]  KbOutMax=[]  KtOutMin=[]  KtOutMax=[]  IntegratorOutMin=[]  IntegratorOutMax=[]  FilterOutMin=[]  FilterOutMax=[]  SumOutMin=[]  SumOutMax=[]  SumI1OutMin=[]  SumI1OutMax=[]  SumI2OutMin=[]  SumI2OutMax=[]  SumI3OutMin=[]  SumI3OutMax=[]  SumDOutMin=[]  SumDOutMax=[]  SaturationOutMin=[]  SaturationOutMax=[]  IntegratorContinuousStateAttributes=''  IntegratorStateMustResolveToSignalObject=off  IntegratorRTWStateStorageClass=Auto  FilterContinuousStateAttributes=''  FilterStateMustResolveToSignalObject=off  FilterRTWStateStorageClass=Auto
  Fast - to -Slow : RateTransition  OutPortSampleTimeMultiple=0.05  OutPortSampleTime=0.1
  Fast - to -Slow1 : RateTransition  OutPortSampleTimeMultiple=0.05  OutPortSampleTime=0.1
  Fast - to -Slow2 : RateTransition  OutPortSampleTimeMultiple=0.05  OutPortSampleTime=0.1
  Gain1 : Gain  Gain=-1
  Scope{1..2,4..9,11..13} (11 alike) : Scope
      Scope1 settings: YMin=-300  YMax=300  SaveName=ScopeData56
      Scope11 settings: YMin=-300  YMax=300  SaveName=ScopeData28
      Scope12 settings: YMin=-300  YMax=300  SaveName=ScopeData30
      Scope13 settings: SaveName=ScopeData31
      Scope2 settings: YMin=-300  YMax=300  SaveName=ScopeData2
      Scope4 settings: YMin=-300  YMax=300  SaveName=ScopeData17
      Scope5 settings: SaveName=ScopeData20
      Scope6 settings: YMin=-300  YMax=300  SaveName=ScopeData18
      Scope7 settings: YMin=-300  YMax=300  SaveName=ScopeData24
      Scope8 settings: TimeRange=10  YMin=-1  YMax=1  SaveName=ScopeData25
      Scope9 settings: SaveName=ScopeData38
  Slow - to - Fast : RateTransition  OutPortSampleTimeMultiple=0.05  OutPortSampleTime=0.05
  Slow - to - Fast1 : RateTransition  OutPortSampleTimeMultiple=0.05  OutPortSampleTime=0.05
  Sum : Sum  Inputs=|+-
  Switch : Switch
  Switch1 : Switch
  gas : Outport
  brake : Outport  Port=2
  wires:
  Discrete Derivative/1 -> Scope8/1, Sum/2
  Discrete PID Controller/1 -> Scope2/1, Scope7/1, Switch/1, Switch/2, Switch1/2, Gain1/1
  Gain1/1 -> Switch1/3
  Switch/1 -> Slow - to - Fast/1, Scope4/1
  Constant/1 -> Switch/3, Switch1/1
  Switch1/1 -> Slow - to - Fast1/1, Scope6/1
  pos/1 -> Scope13/1, Fast - to -Slow/1
  Sum/1 -> Discrete PID Controller/1, Scope9/1
  Fast - to -Slow/1 -> Discrete Derivative/1, Scope5/1
  Slow - to - Fast/1 -> Scope11/1, gas/1
  Slow - to - Fast1/1 -> Scope12/1, brake/1
  Constant2/1 -> Fast - to -Slow1/1
  Fast - to -Slow1/1 -> Sum/1
  Constant1/1 -> Fast - to -Slow2/1
  Fast - to -Slow2/1 -> Discrete PID Controller1/1
  Discrete PID Controller1/1 -> Scope1/1

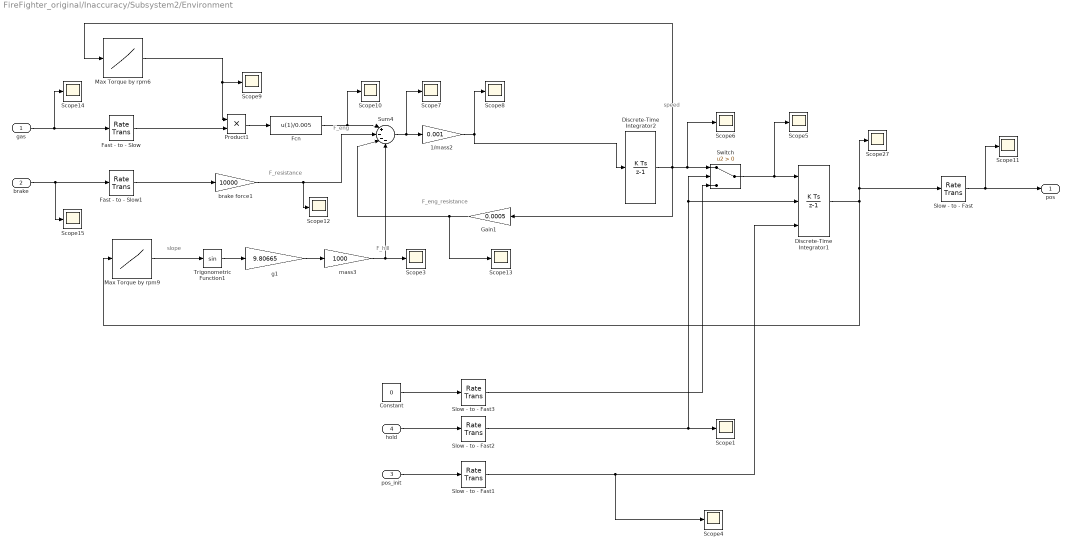
== system FireFighter_original/Inaccuracy/Subsystem2/Environment ==
  note: F_hill
  note: F_eng_resistance
  note: F_resistance
  note: F_eng
  note: speed
  note: slope
  gas : Inport
  brake : Inport  Port=2
  pos_init : Inport  Port=3
  hold : Inport  Port=4
  1/mass2 : Gain  Gain=0.001
  Constant : Constant  Value=0
  Discrete-Time Integrator1 : DiscreteIntegrator  ExternalReset=rising  InitialConditionSource=external  SampleTime=-1  ICPrevOutput=DiscIntNeverNeededParam  ICPrevScaledInput=DiscIntNeverNeededParam
  Discrete-Time Integrator2 : DiscreteIntegrator  SampleTime=-1  ICPrevOutput=DiscIntNeverNeededParam  ICPrevScaledInput=DiscIntNeverNeededParam
  Fast - to - Slow : RateTransition  OutPortSampleTimeMultiple=0.05  OutPortSampleTime=0.1
  "Fast - to - Slow1 " : RateTransition  OutPortSampleTimeMultiple=0.05  OutPortSampleTime=0.1
  Fcn : Fcn  Expr=u(1)/0.005
  Gain1 : Gain  Gain=0.0005
  Max Torque by rpm6 : Lookup_n-D  NumberOfTableDimensions=1  BreakpointsForDimension1=[0;8;20;28;40;60;80;100;120;140;160;180;200]  Table=[165;180;180;170;170;150;115;97;80;70;60;50;40]  RndMeth=Simplest  InputSameDT=on
  Max Torque by rpm9 : Lookup_n-D  NumberOfTableDimensions=1  BreakpointsForDimension1=[0:1000:15000]  Table=[0;pi/60;pi/30;pi/20;pi/15;pi/12;0;0;-pi/18;-pi/36;0;0;0;0;0;0]  RndMeth=Simplest  InputSameDT=on
  Product1 : Product  RndMeth=Zero
  Scope{1,3..15,27} (15 alike) : Scope
      Scope1 settings: TimeRange=10  YMin=-50  YMax=300  SaveName=ScopeData3
      Scope10 settings: SaveName=ScopeData23
      Scope11 settings: TimeRange=10  YMin=-50  YMax=300  SaveName=ScopeData26
      Scope12 settings: SaveName=ScopeData32
      Scope13 settings: SaveName=ScopeData33
      Scope14 settings: SaveName=ScopeData15
      Scope15 settings: SaveName=ScopeData19
      Scope27 settings: TimeRange=10  YMin=2000  YMax=3600  SaveName=ScopeData49
      Scope3 settings: SaveName=ScopeData8
      Scope4 settings: TimeRange=10  YMin=-50  YMax=300  SaveName=ScopeData13
      Scope5 settings: TimeRange=10  YMin=-50  YMax=300  SaveName=ScopeData50
      Scope6 settings: TimeRange=100  YMin=89.9904  YMax=89.9913  SaveName=ScopeData16
      Scope7 settings: SaveName=ScopeData10
      Scope8 settings: SaveName=ScopeData21
      Scope9 settings: SaveName=ScopeData22
  Slow - to - Fast{,1..3} (4 alike) : RateTransition  OutPortSampleTimeMultiple=0.05  OutPortSampleTime=0.05
  Sum4 : Sum  Inputs=|+---
  Switch : Switch  Criteria=u2 > Threshold
  Trigonometric Function1 : Trigonometry
  brake force1 : Gain  Gain=10000
  g1 : Gain  Gain=9.80665
  mass3 : Gain  Gain=1000
  pos : Outport
  wires:
  Product1/1 -> Fcn/1
  brake force1/1 -> Scope12/1, Sum4/2
  Sum4/1 -> Scope7/1, 1/mass2/1
  Gain1/1 -> Sum4/3, Scope13/1
  gas/1 -> Scope14/1, Fast - to - Slow/1
  brake/1 -> Scope15/1, "Fast - to - Slow1 "/1
  Discrete-Time Integrator2/1 -> Max Torque by rpm6/1, Scope6/1, Switch/1, Gain1/1
  Max Torque by rpm9/1 -> Trigonometric Function1/1
  g1/1 -> mass3/1
  Trigonometric Function1/1 -> g1/1
  mass3/1 -> Sum4/4, Scope3/1
  Fcn/1 -> Scope10/1, Sum4/1
  Fast - to - Slow/1 -> Product1/2
  "Fast - to - Slow1 "/1 -> brake force1/1
  Discrete-Time Integrator1/1 -> Scope27/1, Slow - to - Fast/1, Max Torque by rpm9/1
  Slow - to - Fast/1 -> pos/1, Scope11/1
  Max Torque by rpm6/1 -> Product1/1, Scope9/1
  pos_init/1 -> Slow - to - Fast1/1
  hold/1 -> Slow - to - Fast2/1
  Slow - to - Fast1/1 -> Scope4/1, Discrete-Time Integrator1/3
  Constant/1 -> Slow - to - Fast3/1
  Slow - to - Fast3/1 -> Switch/3
  Switch/1 -> Scope5/1, Discrete-Time Integrator1/1
  Slow - to - Fast2/1 -> Switch/2, Discrete-Time Integrator1/2, Scope1/1
  1/mass2/1 -> Scope8/1, Discrete-Time Integrator2/1

== system FireFighter_original/Inaccuracy/Subsystem2/FireFighter ==
  note: current speed
  note: speed=90
  pos : Inport
  Constant : Constant  Value=0
  Constant1 : Constant  Value=0
  Constant2 : Constant  Value=0
  Discrete Derivative : simulink/Discrete/Discrete Derivative  gainval=1.0  ICPrevScaledInput=0.0  InputProcessing=Inherited  OutMin=[]  OutMax=[]  OutDataType=fixdt(1, 16)  OutScaling=2^-10  DoSatur=off
  Discrete PID Controller : simulink/Continuous/PID Controller  Controller=PI  TimeDomain=Discrete-time  SampleTime=-1  IntegratorMethod=Forward Euler  FilterMethod=Forward Euler  Form=Parallel  P=0.05  I=0.000228325  D=0  N=100  InitialConditionSource=internal  InitialConditionForIntegrator=0  InitialConditionForFilter=0  ExternalReset=none  LimitOutput=on  UpperSaturationLimit=1  LowerSaturationLimit=-1  LinearizeAsGain=off  AntiWindupMode=back-calculation  Kb=0.01  TrackingMode=off  Kt=1  PParamMin=[]  PParamMax=[]  IParamMin=[]  IParamMax=[]  DParamMin=[]  DParamMax=[]  NParamMin=[]  NParamMax=[]  KbParamMin=[]  KbParamMax=[]  KtParamMin=[]  KtParamMax=[]  POutMin=[]  POutMax=[]  IOutMin=[]  IOutMax=[]  DOutMin=[]  DOutMax=[]  NOutMin=[]  NOutMax=[]  KbOutMin=[]  KbOutMax=[]  KtOutMin=[]  KtOutMax=[]  IntegratorOutMin=[]  IntegratorOutMax=[]  FilterOutMin=[]  FilterOutMax=[]  SumOutMin=[]  SumOutMax=[]  SumI1OutMin=[]  SumI1OutMax=[]  SumI2OutMin=[]  SumI2OutMax=[]  SumI3OutMin=[]  SumI3OutMax=[]  SumDOutMin=[]  SumDOutMax=[]  SaturationOutMin=[]  SaturationOutMax=[]  IntegratorContinuousStateAttributes=''  IntegratorStateMustResolveToSignalObject=off  IntegratorRTWStateStorageClass=Auto  FilterContinuousStateAttributes=''  FilterStateMustResolveToSignalObject=off  FilterRTWStateStorageClass=Auto
  Discrete PID Controller1 : simulink/Continuous/PID Controller  Controller=PI  TimeDomain=Discrete-time  SampleTime=-1  IntegratorMethod=Forward Euler  FilterMethod=Forward Euler  Form=Parallel  P=0.05  I=0.000228325  D=0  N=100  InitialConditionSource=internal  InitialConditionForIntegrator=0  InitialConditionForFilter=0  ExternalReset=none  LimitOutput=on  UpperSaturationLimit=1  LowerSaturationLimit=-1  LinearizeAsGain=off  AntiWindupMode=back-calculation  Kb=0.01  TrackingMode=off  Kt=1  PParamMin=[]  PParamMax=[]  IParamMin=[]  IParamMax=[]  DParamMin=[]  DParamMax=[]  NParamMin=[]  NParamMax=[]  KbParamMin=[]  KbParamMax=[]  KtParamMin=[]  KtParamMax=[]  POutMin=[]  POutMax=[]  IOutMin=[]  IOutMax=[]  DOutMin=[]  DOutMax=[]  NOutMin=[]  NOutMax=[]  KbOutMin=[]  KbOutMax=[]  KtOutMin=[]  KtOutMax=[]  IntegratorOutMin=[]  IntegratorOutMax=[]  FilterOutMin=[]  FilterOutMax=[]  SumOutMin=[]  SumOutMax=[]  SumI1OutMin=[]  SumI1OutMax=[]  SumI2OutMin=[]  SumI2OutMax=[]  SumI3OutMin=[]  SumI3OutMax=[]  SumDOutMin=[]  SumDOutMax=[]  SaturationOutMin=[]  SaturationOutMax=[]  IntegratorContinuousStateAttributes=''  IntegratorStateMustResolveToSignalObject=off  IntegratorRTWStateStorageClass=Auto  FilterContinuousStateAttributes=''  FilterStateMustResolveToSignalObject=off  FilterRTWStateStorageClass=Auto
  Fast - to -Slow : RateTransition  OutPortSampleTimeMultiple=0.05  OutPortSampleTime=0.1
  Fast - to -Slow1 : RateTransition  OutPortSampleTimeMultiple=0.05  OutPortSampleTime=0.1
  Fast - to -Slow2 : RateTransition  OutPortSampleTimeMultiple=0.05  OutPortSampleTime=0.1
  Gain1 : Gain  Gain=-1
  Scope{1..2,4..9,11..13} (11 alike) : Scope
      Scope1 settings: YMin=-300  YMax=300  SaveName=ScopeData52
      Scope11 settings: YMin=-300  YMax=300  SaveName=ScopeData28
      Scope12 settings: YMin=-300  YMax=300  SaveName=ScopeData30
      Scope13 settings: SaveName=ScopeData31
      Scope2 settings: YMin=-300  YMax=300  SaveName=ScopeData2
      Scope4 settings: YMin=-300  YMax=300  SaveName=ScopeData17
      Scope5 settings: SaveName=ScopeData20
      Scope6 settings: YMin=-300  YMax=300  SaveName=ScopeData18
      Scope7 settings: YMin=-300  YMax=300  SaveName=ScopeData24
      Scope8 settings: TimeRange=10  SaveName=ScopeData25
      Scope9 settings: SaveName=ScopeData38
  Slow - to - Fast : RateTransition  OutPortSampleTimeMultiple=0.05  OutPortSampleTime=0.05
  Slow - to - Fast1 : RateTransition  OutPortSampleTimeMultiple=0.05  OutPortSampleTime=0.05
  Sum : Sum  Inputs=|+-
  Switch : Switch
  Switch1 : Switch
  gas : Outport
  brake : Outport  Port=2
  wires:
  Discrete Derivative/1 -> Scope8/1, Sum/2
  Discrete PID Controller/1 -> Scope2/1, Scope7/1, Switch/1, Switch/2, Switch1/2, Gain1/1
  Gain1/1 -> Switch1/3
  Switch/1 -> Slow - to - Fast/1, Scope4/1
  Constant/1 -> Switch/3, Switch1/1
  Switch1/1 -> Slow - to - Fast1/1, Scope6/1
  pos/1 -> Scope13/1, Fast - to -Slow/1
  Sum/1 -> Discrete PID Controller/1, Scope9/1
  Fast - to -Slow/1 -> Discrete Derivative/1, Scope5/1
  Slow - to - Fast/1 -> Scope11/1, gas/1
  Slow - to - Fast1/1 -> Scope12/1, brake/1
  Constant2/1 -> Fast - to -Slow1/1
  Fast - to -Slow1/1 -> Sum/1
  Discrete PID Controller1/1 -> Scope1/1
  Constant1/1 -> Fast - to -Slow2/1
  Fast - to -Slow2/1 -> Discrete PID Controller1/1

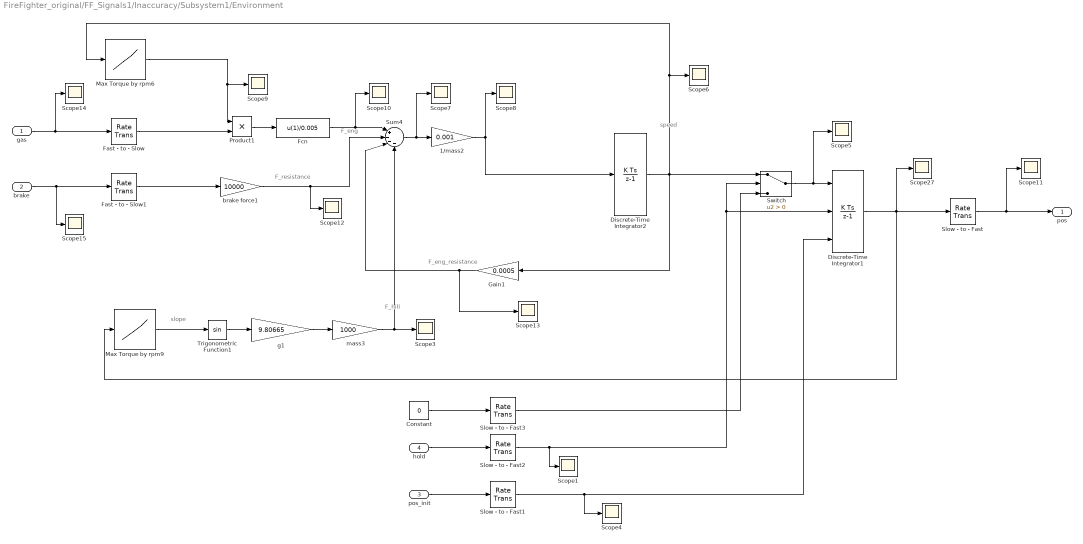
== system FireFighter_original/FF_Signals1/Inaccuracy/Subsystem1/Environment ==
  note: F_hill
  note: F_eng_resistance
  note: F_resistance
  note: F_eng
  note: slope
  note: speed
  gas : Inport
  brake : Inport  Port=2
  pos_init : Inport  Port=3
  hold : Inport  Port=4
  1/mass2 : Gain  Gain=0.001
  Constant : Constant  Value=0
  Discrete-Time Integrator1 : DiscreteIntegrator  ExternalReset=rising  InitialConditionSource=external  SampleTime=-1  ICPrevOutput=DiscIntNeverNeededParam  ICPrevScaledInput=DiscIntNeverNeededParam
  Discrete-Time Integrator2 : DiscreteIntegrator  SampleTime=-1  ICPrevOutput=DiscIntNeverNeededParam  ICPrevScaledInput=DiscIntNeverNeededParam
  Fast - to - Slow : RateTransition  OutPortSampleTimeMultiple=0.05  OutPortSampleTime=0.1
  "Fast - to - Slow1 " : RateTransition  OutPortSampleTimeMultiple=0.05  OutPortSampleTime=0.1
  Fcn : Fcn  Expr=u(1)/0.005
  Gain1 : Gain  Gain=0.0005
  Max Torque by rpm6 : Lookup_n-D  NumberOfTableDimensions=1  BreakpointsForDimension1=[0;8;20;28;40;60;80;100;120;140;160;180;200]  Table=[165;180;180;170;170;150;115;97;80;70;60;50;40]  RndMeth=Simplest  InputSameDT=on
  Max Torque by rpm9 : Lookup_n-D  NumberOfTableDimensions=1  BreakpointsForDimension1=[0:1000:15000]  Table=[0;pi/60;pi/30;pi/20;pi/15;pi/12;0;0;-pi/18;-pi/36;0;0;0;0;0;0]  RndMeth=Simplest  InputSameDT=on
  Product1 : Product  RndMeth=Zero
  Scope{1,3..15,27} (15 alike) : Scope
      Scope1 settings: TimeRange=10  YMin=-50  YMax=300  SaveName=ScopeData51
      Scope10 settings: SaveName=ScopeData23
      Scope11 settings: TimeRange=10  YMin=-50  YMax=300  SaveName=ScopeData26
      Scope12 settings: SaveName=ScopeData32
      Scope13 settings: SaveName=ScopeData33
      Scope14 settings: SaveName=ScopeData15
      Scope15 settings: SaveName=ScopeData19
      Scope27 settings: TimeRange=10  YMin=-50  YMax=300  SaveName=ScopeData49
      Scope3 settings: SaveName=ScopeData8
      Scope4 settings: TimeRange=10  YMin=-50  YMax=300  SaveName=ScopeData53
      Scope5 settings: TimeRange=10  YMin=-50  YMax=300  SaveName=ScopeData54
      Scope6 settings: TimeRange=100  YMin=0  YMax=300  SaveName=ScopeData55
      Scope7 settings: SaveName=ScopeData10
      Scope8 settings: SaveName=ScopeData21
      Scope9 settings: SaveName=ScopeData22
  Slow - to - Fast{,1..3} (4 alike) : RateTransition  OutPortSampleTimeMultiple=0.05  OutPortSampleTime=0.05
  Sum4 : Sum  Inputs=|+---
  Switch : Switch  Criteria=u2 > Threshold
  Trigonometric Function1 : Trigonometry
  brake force1 : Gain  Gain=10000
  g1 : Gain  Gain=9.80665
  mass3 : Gain  Gain=1000
  pos : Outport
  wires:
  Product1/1 -> Fcn/1
  brake force1/1 -> Scope12/1, Sum4/2
  Sum4/1 -> Scope7/1, 1/mass2/1
  1/mass2/1 -> Discrete-Time Integrator2/1, Scope8/1
  Gain1/1 -> Scope13/1, Sum4/3
  gas/1 -> Scope14/1, Fast - to - Slow/1
  brake/1 -> Scope15/1, "Fast - to - Slow1 "/1
  Max Torque by rpm9/1 -> Trigonometric Function1/1
  g1/1 -> mass3/1
  Trigonometric Function1/1 -> g1/1
  mass3/1 -> Sum4/4, Scope3/1
  Fcn/1 -> Scope10/1, Sum4/1
  Fast - to - Slow/1 -> Product1/2
  "Fast - to - Slow1 "/1 -> brake force1/1
  Slow - to - Fast/1 -> pos/1, Scope11/1
  Max Torque by rpm6/1 -> Product1/1, Scope9/1
  Discrete-Time Integrator2/1 -> Max Torque by rpm6/1, Scope6/1, Switch/1, Gain1/1
  pos_init/1 -> Slow - to - Fast1/1
  hold/1 -> Slow - to - Fast2/1
  Slow - to - Fast2/1 -> Switch/2, Discrete-Time Integrator1/2, Scope1/1
  Slow - to - Fast1/1 -> Scope4/1, Discrete-Time Integrator1/3
  Constant/1 -> Slow - to - Fast3/1
  Slow - to - Fast3/1 -> Switch/3
  Discrete-Time Integrator1/1 -> Max Torque by rpm9/1, Scope27/1, Slow - to - Fast/1
  Switch/1 -> Scope5/1, Discrete-Time Integrator1/1

== system FireFighter_original/FF_Signals1/Inaccuracy/Subsystem1/FireFighter ==
  note: current speed
  note: speed=90
  pos : Inport
  Constant : Constant  Value=0
  Constant1 : Constant  Value=250
  Constant2 : Constant  Value=250
  Discrete Derivative : simulink/Discrete/Discrete Derivative  gainval=1.0  ICPrevScaledInput=0.0  InputProcessing=Inherited  OutMin=[]  OutMax=[]  OutDataType=fixdt(1, 16)  OutScaling=2^-10  DoSatur=off
  Discrete PID Controller : simulink/Continuous/PID Controller  Controller=PI  TimeDomain=Discrete-time  SampleTime=-1  IntegratorMethod=Forward Euler  FilterMethod=Forward Euler  Form=Parallel  P=0.05  I=0.000228325  D=0  N=100  InitialConditionSource=internal  InitialConditionForIntegrator=0  InitialConditionForFilter=0  ExternalReset=none  LimitOutput=on  UpperSaturationLimit=1  LowerSaturationLimit=-1  LinearizeAsGain=off  AntiWindupMode=back-calculation  Kb=0.01  TrackingMode=off  Kt=1  PParamMin=[]  PParamMax=[]  IParamMin=[]  IParamMax=[]  DParamMin=[]  DParamMax=[]  NParamMin=[]  NParamMax=[]  KbParamMin=[]  KbParamMax=[]  KtParamMin=[]  KtParamMax=[]  POutMin=[]  POutMax=[]  IOutMin=[]  IOutMax=[]  DOutMin=[]  DOutMax=[]  NOutMin=[]  NOutMax=[]  KbOutMin=[]  KbOutMax=[]  KtOutMin=[]  KtOutMax=[]  IntegratorOutMin=[]  IntegratorOutMax=[]  FilterOutMin=[]  FilterOutMax=[]  SumOutMin=[]  SumOutMax=[]  SumI1OutMin=[]  SumI1OutMax=[]  SumI2OutMin=[]  SumI2OutMax=[]  SumI3OutMin=[]  SumI3OutMax=[]  SumDOutMin=[]  SumDOutMax=[]  SaturationOutMin=[]  SaturationOutMax=[]  IntegratorContinuousStateAttributes=''  IntegratorStateMustResolveToSignalObject=off  IntegratorRTWStateStorageClass=Auto  FilterContinuousStateAttributes=''  FilterStateMustResolveToSignalObject=off  FilterRTWStateStorageClass=Auto
  Discrete PID Controller1 : simulink/Continuous/PID Controller  Controller=PI  TimeDomain=Discrete-time  SampleTime=-1  IntegratorMethod=Forward Euler  FilterMethod=Forward Euler  Form=Parallel  P=0.05  I=0.000228325  D=0  N=100  InitialConditionSource=internal  InitialConditionForIntegrator=0  InitialConditionForFilter=0  ExternalReset=none  LimitOutput=on  UpperSaturationLimit=1  LowerSaturationLimit=-1  LinearizeAsGain=off  AntiWindupMode=back-calculation  Kb=0.01  TrackingMode=off  Kt=1  PParamMin=[]  PParamMax=[]  IParamMin=[]  IParamMax=[]  DParamMin=[]  DParamMax=[]  NParamMin=[]  NParamMax=[]  KbParamMin=[]  KbParamMax=[]  KtParamMin=[]  KtParamMax=[]  POutMin=[]  POutMax=[]  IOutMin=[]  IOutMax=[]  DOutMin=[]  DOutMax=[]  NOutMin=[]  NOutMax=[]  KbOutMin=[]  KbOutMax=[]  KtOutMin=[]  KtOutMax=[]  IntegratorOutMin=[]  IntegratorOutMax=[]  FilterOutMin=[]  FilterOutMax=[]  SumOutMin=[]  SumOutMax=[]  SumI1OutMin=[]  SumI1OutMax=[]  SumI2OutMin=[]  SumI2OutMax=[]  SumI3OutMin=[]  SumI3OutMax=[]  SumDOutMin=[]  SumDOutMax=[]  SaturationOutMin=[]  SaturationOutMax=[]  IntegratorContinuousStateAttributes=''  IntegratorStateMustResolveToSignalObject=off  IntegratorRTWStateStorageClass=Auto  FilterContinuousStateAttributes=''  FilterStateMustResolveToSignalObject=off  FilterRTWStateStorageClass=Auto
  Fast - to -Slow : RateTransition  OutPortSampleTimeMultiple=0.05  OutPortSampleTime=0.1
  Fast - to -Slow1 : RateTransition  OutPortSampleTimeMultiple=0.05  OutPortSampleTime=0.1
  Fast - to -Slow2 : RateTransition  OutPortSampleTimeMultiple=0.05  OutPortSampleTime=0.1
  Gain1 : Gain  Gain=-1
  Scope{1..2,4..9,11..13} (11 alike) : Scope
      Scope1 settings: YMin=-300  YMax=300  SaveName=ScopeData56
      Scope11 settings: YMin=-300  YMax=300  SaveName=ScopeData28
      Scope12 settings: YMin=-300  YMax=300  SaveName=ScopeData30
      Scope13 settings: SaveName=ScopeData31
      Scope2 settings: YMin=-300  YMax=300  SaveName=ScopeData2
      Scope4 settings: YMin=-300  YMax=300  SaveName=ScopeData17
      Scope5 settings: SaveName=ScopeData20
      Scope6 settings: YMin=-300  YMax=300  SaveName=ScopeData18
      Scope7 settings: YMin=-300  YMax=300  SaveName=ScopeData24
      Scope8 settings: TimeRange=10  YMin=-1  YMax=1  SaveName=ScopeData25
      Scope9 settings: SaveName=ScopeData38
  Slow - to - Fast : RateTransition  OutPortSampleTimeMultiple=0.05  OutPortSampleTime=0.05
  Slow - to - Fast1 : RateTransition  OutPortSampleTimeMultiple=0.05  OutPortSampleTime=0.05
  Sum : Sum  Inputs=|+-
  Switch : Switch
  Switch1 : Switch
  gas : Outport
  brake : Outport  Port=2
  wires:
  Discrete Derivative/1 -> Scope8/1, Sum/2
  Discrete PID Controller/1 -> Scope2/1, Scope7/1, Switch/1, Switch/2, Switch1/2, Gain1/1
  Gain1/1 -> Switch1/3
  Switch/1 -> Slow - to - Fast/1, Scope4/1
  Constant/1 -> Switch/3, Switch1/1
  Switch1/1 -> Slow - to - Fast1/1, Scope6/1
  pos/1 -> Scope13/1, Fast - to -Slow/1
  Sum/1 -> Discrete PID Controller/1, Scope9/1
  Fast - to -Slow/1 -> Discrete Derivative/1, Scope5/1
  Slow - to - Fast/1 -> Scope11/1, gas/1
  Slow - to - Fast1/1 -> Scope12/1, brake/1
  Constant2/1 -> Fast - to -Slow1/1
  Fast - to -Slow1/1 -> Sum/1
  Constant1/1 -> Fast - to -Slow2/1
  Fast - to -Slow2/1 -> Discrete PID Controller1/1
  Discrete PID Controller1/1 -> Scope1/1
